simulink model "test_model"  (R2020a)
settings: Solver=FixedStepDiscrete  StartTime=0.0  StopTime=10.0  FixedStep=0.01  RelTol=1e-3
undefined symbols (not defined in the file): judge_val, output_val
settings Model: Creator=1014721  LastModifiedBy=1014721
settings OptimizationCC: DefaultParameterBehavior=Inlined  EnhancedBackFolding=on  PassReuseOutputArgsAs=Individual arguments  ZeroExternalMemoryAtStartup=off  ZeroInternalMemoryAtStartup=off  OptimizeBlockOrder=speed  DifferentSizesBufferReuse=on  OptimizationCustomize=off  EfficientTunableParamExpr=on
settings DebuggingCC: ParameterTunabilityLossMsg=error
settings SFSimCC: MATLABDynamicMemAlloc=off
settings RTWCC: SystemTargetFile=ert.tlc  GenCodeOnly=on  TemplateMakefile=ert_default_tmf  GenerateReport=on  LaunchReport=on
settings CodeAppCC: ForceParamTrailComments=on  IgnoreCustomStorageClasses=off  OperatorAnnotations=on  SimulinkDataObjDesc=on  SFDataObjDesc=on  InsertBlockDesc=on
settings ERTTargetCC: TargetLangStandard=C99 (ISO)  GenerateSampleERTMain=on  InlinedParameterPlacement=NonHierarchical  ERTCustomFileTemplate=example_file_process.tlc

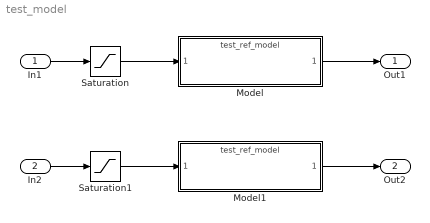
== system test_model ==
  In1 : Inport
  In2 : Inport  Port=2
  Model : ModelReference  ModelNameDialog=test_ref_model.slx  ParameterArgumentNames=judge_val,output_val  ParameterArgumentValues=judge_val,output_val  UsingDefaultArgumentValue=0,0  SimulationMode=Normal  ModelReferenceVersion=1.11  judge_val=10  output_val=1  SimulationMode=Normal
  Model1 : ModelReference  ModelNameDialog=test_ref_model.slx  ParameterArgumentNames=judge_val,output_val  ParameterArgumentValues=judge_val,output_val  UsingDefaultArgumentValue=0,0  SimulationMode=Normal  ModelReferenceVersion=1.11  judge_val=10  output_val=1  SimulationMode=Normal
  Saturation : Saturate  UpperLimit=20  LowerLimit=-20
      settings: AttributesFormatString=|
      | 上限：%<UpperLimit>
      | 下限：%<LowerLimit>
  Saturation1 : Saturate  UpperLimit=5  LowerLimit=-5
      settings: AttributesFormatString=|
      | 上限：%<UpperLimit>
      | 下限：%<LowerLimit>
  Out1 : Outport
  Out2 : Outport  Port=2
  wires:
  In1/1 -> Saturation/1
  Model/1 -> Out1/1
  Saturation/1 -> Model/1
  Saturation1/1 -> Model1/1
  In2/1 -> Saturation1/1
  Model1/1 -> Out2/1
